simulink model "SF007A_SysFricLrng"  (R2013b)
settings: Solver=FixedStepDiscrete  SolverMode=SingleTasking  StartTime=0.0  StopTime=1  FixedStep=0.002  RelTol=1e-3
PostLoadFcn:
  | , if any(exist('dsrtsu_mdlpostloadfcn', 'file') == [2, 3, 6]), try dsrtsu_mdlpostloadfcn('Execute', bdroot); catch fprintf('Error in PostLoadFcn (dsrtsu_mdlpostloadfcn) for model "%s":\n %s\n', bdroot, lasterr); end, end,
undefined symbols (not defined in the file): ARCHGLBPRM_100MILLISEC_SEC_F32, ARCHGLBPRM_10MILLISEC_SEC_F32, ARCHGLBPRM_180OVERPI_ULS_F32, CONV100MICROSECTOSEC_ULS_F32, FLTINJ_SYSFRICLRNG_SYSFRICOFFS, FricLrngData, HiFricNtc, HWPTNUM_CNT_U08, HWPTNUMSUB1_CNT_U08, HWVELDECDIR_ULS_U08, HWVELINCDIR_ULS_U08, IDXCALCNSCAGFAC_ULS_U08, IDXSELN1_ULS_U08, IDXSELN2_ULS_U08, IDXSELN3_ULS_U08, LRNGENASCAFAC_MILLISEC_U32, NtcSts1, SCAGFACQUARTER_CNT_F32, SCAGFACTEN_CNT_U16, SECIDXSELN_ULS_U08, SysFricLrngBasLineEolFric, SysFricLrngBasLineFric, SysFricLrngBasLineHys, SysFricLrngBasLineRngCntr, SysFricLrngEolFricDifScagFac, SysFricLrngFricChgWght, SysFricLrngFricDiagcThd, SysFricLrngFricDiagcTiThd, SysFricLrngFricHysHwAgPt, SysFricLrngGain, SysFricLrngHwPosnAuthyThd, SysFricLrngHwVelConstrLim, SysFricLrngHwVelHiLim, SysFricLrngHwVelLoLim, SysFricLrngIgnCycFricChgLim, SysFricLrngLatAHiLim, SysFricLrngLatALoLim, SysFricLrngMaskVehSpd, SysFricLrngOperMod1, SysFricLrngRngCntrThd, SysFricLrngThd, SysFricLrngTHiLim, SysFricLrngTLoLim, SysFricLrngVehSpd, SYSFRICOFFSLIM_HWNWTMTR_F32, VEHSPDPTNUM1_ULS_U08, VEHSPDPTNUM2_ULS_U08
libraries: Fil x19, simulink x17, NxtrLim x10, NxtrAbslt x3, NxtrNvM x2, FixdToFloat x2, FloatToFixd x1, LnrIntrpn x1
(part 7 of 7)

== system SF007A_SysFricLrng/SysFricLrng/SysFricLrngPer1/RunningAndCalibrationModes/FricLearning/Calculate Average Friction/Raw Average Calculation/Update LPF/InitAvrgFricLpFil1 ==
  RawAvgFric : Inport
  Action Port : ActionPort  ActionType=case
  CopyRight2 : Subsystem  Description=|  mask(Copyright Information){none=on}
      | Copyright info block.                                               
      |                                                                     
      | Place copyright information at the top of every subsystem in design.
      mask prompts: none "No parameters"
      mask help: Place copyright information at the top of every subsystem in design.
      mask Display:
      | NxtrConf = 'Nexteer Confidential';
      | 
      | sys = bdroot; %handle for the current model ("system")
      | first = get_param(sys,'Created');
      | first = first(end-3:end);  %year is last four digits
      | 
      | last = get_param(sys,'LastModifiedDate');
      | if isempty(last)
      |     last = datestr(now,'yyyy');
      | else
      |     last = last(end-3:end);
      | end
      | 
      | if strcmp(first,last)
      |     fprintf('%s -- Copyright %s Nexteer',NxtrConf,first)
      | else
      |     fprintf('%s -- %s%s- %s Nexteer',NxtrConf,char(169),first,last)
      | end
  FilLpUpdOutp : Subsystem  mask(FilLpUpdOutp){StVar=AvrgFricLpFil1}
      mask prompts: StVar "State Variable:"
      mask help: Simulink implementation of the LPF_OpUpdate_f32_m macro.
      mask init: same as SF007A_SysFricLrng/SysFricLrng/SysFricLrngPer1/RunningAndCalibrationModes/Running Mode/If Action Subsystem/BlendingFricChg/FilLpUpdOutp
      settings: AttributesFormatString=StVar: %<StVar>
      mask Display:
      | port_label('input',1,'Inp')
      | port_label('output',1,'Outp')
      | text(0.2,0.8,'FilLpUpdOutp')
  FiltAvgFric : Outport
  wires:
  RawAvgFric/1 -> FilLpUpdOutp/1(Input)
  FilLpUpdOutp/1(Out1) -> FiltAvgFric/1

== system SF007A_SysFricLrng/SysFricLrng/SysFricLrngPer1/RunningAndCalibrationModes/FricLearning/Calculate Average Friction/Raw Average Calculation/Update LPF/InitAvrgFricLpFil2 ==
  RawAvgFric : Inport
  Action Port : ActionPort  ActionType=case
  CopyRight2 : Subsystem  Description=|  mask(Copyright Information){none=on}
      | Copyright info block.                                               
      |                                                                     
      | Place copyright information at the top of every subsystem in design.
      mask prompts: none "No parameters"
      mask help: Place copyright information at the top of every subsystem in design.
      mask Display:
      | NxtrConf = 'Nexteer Confidential';
      | 
      | sys = bdroot; %handle for the current model ("system")
      | first = get_param(sys,'Created');
      | first = first(end-3:end);  %year is last four digits
      | 
      | last = get_param(sys,'LastModifiedDate');
      | if isempty(last)
      |     last = datestr(now,'yyyy');
      | else
      |     last = last(end-3:end);
      | end
      | 
      | if strcmp(first,last)
      |     fprintf('%s -- Copyright %s Nexteer',NxtrConf,first)
      | else
      |     fprintf('%s -- %s%s- %s Nexteer',NxtrConf,char(169),first,last)
      | end
  FilLpUpdOutp : Subsystem  mask(FilLpUpdOutp){StVar=AvrgFricLpFil2}
      mask prompts: StVar "State Variable:"
      mask help: Simulink implementation of the LPF_OpUpdate_f32_m macro.
      mask init: same as SF007A_SysFricLrng/SysFricLrng/SysFricLrngPer1/RunningAndCalibrationModes/Running Mode/If Action Subsystem/BlendingFricChg/FilLpUpdOutp
      settings: AttributesFormatString=StVar: %<StVar>
      mask Display:
      | port_label('input',1,'Inp')
      | port_label('output',1,'Outp')
      | text(0.2,0.8,'FilLpUpdOutp')
  FiltAvgFric : Outport
  wires:
  RawAvgFric/1 -> FilLpUpdOutp/1(Input)
  FilLpUpdOutp/1(Out1) -> FiltAvgFric/1

== system SF007A_SysFricLrng/SysFricLrng/SysFricLrngPer1/RunningAndCalibrationModes/FricLearning/Calculate Average Friction/Raw Average Calculation/Update LPF/InitAvrgFricLpFil3 ==
  RawAvgFric : Inport
  Action Port : ActionPort  ActionType=case
  CopyRight2 : Subsystem  Description=|  mask(Copyright Information){none=on}
      | Copyright info block.                                               
      |                                                                     
      | Place copyright information at the top of every subsystem in design.
      mask prompts: none "No parameters"
      mask help: Place copyright information at the top of every subsystem in design.
      mask Display:
      | NxtrConf = 'Nexteer Confidential';
      | 
      | sys = bdroot; %handle for the current model ("system")
      | first = get_param(sys,'Created');
      | first = first(end-3:end);  %year is last four digits
      | 
      | last = get_param(sys,'LastModifiedDate');
      | if isempty(last)
      |     last = datestr(now,'yyyy');
      | else
      |     last = last(end-3:end);
      | end
      | 
      | if strcmp(first,last)
      |     fprintf('%s -- Copyright %s Nexteer',NxtrConf,first)
      | else
      |     fprintf('%s -- %s%s- %s Nexteer',NxtrConf,char(169),first,last)
      | end
  FilLpUpdOutp : Subsystem  mask(FilLpUpdOutp){StVar=AvrgFricLpFil3}
      mask prompts: StVar "State Variable:"
      mask help: Simulink implementation of the LPF_OpUpdate_f32_m macro.
      mask init: same as SF007A_SysFricLrng/SysFricLrng/SysFricLrngPer1/RunningAndCalibrationModes/Running Mode/If Action Subsystem/BlendingFricChg/FilLpUpdOutp
      settings: AttributesFormatString=StVar: %<StVar>
      mask Display:
      | port_label('input',1,'Inp')
      | port_label('output',1,'Outp')
      | text(0.2,0.8,'FilLpUpdOutp')
  FiltAvgFric : Outport
  wires:
  RawAvgFric/1 -> FilLpUpdOutp/1(Input)
  FilLpUpdOutp/1(Out1) -> FiltAvgFric/1

== system SF007A_SysFricLrng/SysFricLrng/SysFricLrngPer1/RunningAndCalibrationModes/FricLearning/Calculate Average Friction/Raw Average Calculation/Update LPF/InitAvrgFricLpFil4 ==
  RawAvgFric : Inport
  Action Port : ActionPort  ActionType=default
  CopyRight2 : Subsystem  Description=|  mask(Copyright Information){none=on}
      | Copyright info block.                                               
      |                                                                     
      | Place copyright information at the top of every subsystem in design.
      mask prompts: none "No parameters"
      mask help: Place copyright information at the top of every subsystem in design.
      mask Display:
      | NxtrConf = 'Nexteer Confidential';
      | 
      | sys = bdroot; %handle for the current model ("system")
      | first = get_param(sys,'Created');
      | first = first(end-3:end);  %year is last four digits
      | 
      | last = get_param(sys,'LastModifiedDate');
      | if isempty(last)
      |     last = datestr(now,'yyyy');
      | else
      |     last = last(end-3:end);
      | end
      | 
      | if strcmp(first,last)
      |     fprintf('%s -- Copyright %s Nexteer',NxtrConf,first)
      | else
      |     fprintf('%s -- %s%s- %s Nexteer',NxtrConf,char(169),first,last)
      | end
  FilLpUpdOutp : Subsystem  mask(FilLpUpdOutp){StVar=AvrgFricLpFil4}
      mask prompts: StVar "State Variable:"
      mask help: Simulink implementation of the LPF_OpUpdate_f32_m macro.
      mask init: same as SF007A_SysFricLrng/SysFricLrng/SysFricLrngPer1/RunningAndCalibrationModes/Running Mode/If Action Subsystem/BlendingFricChg/FilLpUpdOutp
      settings: AttributesFormatString=StVar: %<StVar>
      mask Display:
      | port_label('input',1,'Inp')
      | port_label('output',1,'Outp')
      | text(0.2,0.8,'FilLpUpdOutp')
  FiltAvgFric : Outport
  wires:
  RawAvgFric/1 -> FilLpUpdOutp/1(Input)
  FilLpUpdOutp/1(Out1) -> FiltAvgFric/1

== system SF007A_SysFricLrng/SysFricLrng/SysFricLrngPer1/RunningAndCalibrationModes/FricLearning/Range Counter Manager/Range Counter Control1/UpdateBaselineFric/CopyRight2 ==

== system SF007A_SysFricLrng/SysFricLrng/SysFricLrngPer1/RunningAndCalibrationModes/FricLearning/Range Counter Manager/Range Counter Threshold Calculation/Do Nothig/CopyRight2 ==

== system SF007A_SysFricLrng/SysFricLrng/SysFricLrngPer1/RunningAndCalibrationModes/FricLearning/Range Counter Manager/Range Counter Threshold Calculation/RangeCounterThreshExceeded/CopyRight2 ==

== system SF007A_SysFricLrng/SysFricLrng/SysFricLrngPer1/RunningAndCalibrationModes/LearningConstraint/ColTqconstraint/ColTqAryCalcn/12 Delay's Execution/CopyRight2 ==

== system SF007A_SysFricLrng/SysFricLrng/SysFricLrngPer1/RunningAndCalibrationModes/LearningConstraint/HwAngConstraint/Handwheel Angle Buffer/12 Delay's Execution/CopyRight2 ==

== system SF007A_SysFricLrng/SysFricLrng/SysFricLrngPer1/RunningAndCalibrationModes/LearningConstraint/HwVelConstraint/Handwheel Velocity Buffer/12 Delay's Execution/CopyRight2 ==

== system SF007A_SysFricLrng/SysFricLrng/SysFricLrngPer1/RunningAndCalibrationModes/LearningConstraint/HwVelConstraint/Range_Monotonicity Calculation/ AllGTZ/CopyRight2 ==

== system SF007A_SysFricLrng/SysFricLrng/SysFricLrngPer1/RunningAndCalibrationModes/LearningConstraint/HwVelConstraint/Range_Monotonicity Calculation/AllLTZ/CopyRight2 ==

== system SF007A_SysFricLrng/SysFricLrng/SysFricLrngPer1/RunningAndCalibrationModes/LearningConstraint/VehSpdConstraint/VehSpdIdxCalcn/If Action Subsystem/CopyRight2 ==

== system SF007A_SysFricLrng/SysFricLrng/SysFricLrngPer1/RunningAndCalibrationModes/LearningConstraint/VehSpdConstraint/VehSpdIdxCalcn/If Action Subsystem1/CopyRight2 ==

== system SF007A_SysFricLrng/SysFricLrng/SysFricLrngPer1/RunningAndCalibrationModes/FricLearning/Calculate Average Friction/NTC FAIL/GetTiSpan100MicroSec32bit/No wrapping/CopyRight2 ==

== system SF007A_SysFricLrng/SysFricLrng/SysFricLrngPer1/RunningAndCalibrationModes/FricLearning/Calculate Average Friction/NTC FAIL/GetTiSpan100MicroSec32bit/Wrapping/CopyRight2 ==

== system SF007A_SysFricLrng/SysFricLrng/SysFricLrngPer1/RunningAndCalibrationModes/FricLearning/Calculate Average Friction/NTC FAIL/NTCFAIL/SetNtcSts/SetNtcSts ==
  note: Note:
      |
      | - "ISO Fault Debounce Design" Simulink block intent to use here for Simulation purpose only. Do not Code this block
  NtcNr : Inport
  NtcStInfo : Inport  Port=2
  NtcSts : Inport  Port=3
  DebStep : Inport  Port=4
  CopyRight2 : Subsystem  Description=|  mask(Copyright Information){none=on}
      | Copyright info block.                                               
      |                                                                     
      | Place copyright information at the top of every subsystem in design.
      mask prompts: none "No parameters"
      mask help: Place copyright information at the top of every subsystem in design.
      mask Display:
      | NxtrConf = 'Nexteer Confidential';
      | 
      | sys = bdroot; %handle for the current model ("system")
      | first = get_param(sys,'Created');
      | first = first(end-3:end);  %year is last four digits
      | 
      | last = get_param(sys,'LastModifiedDate');
      | if isempty(last)
      |     last = datestr(now,'yyyy');
      | else
      |     last = last(end-3:end);
      | end
      | 
      | if strcmp(first,last)
      |     fprintf('%s -- Copyright %s Nexteer',NxtrConf,first)
      | else
      |     fprintf('%s -- %s%s- %s Nexteer',NxtrConf,char(169),first,last)
      | end
  Data Store Write : DataStoreWrite  DataStoreName=Ntc0X0A2Qlfr
  Data Type Conversion4 : DataTypeConversion  OutDataTypeStr=Enum: SigQlfr1
  Ground : Ground
  ISO Fault Debounce Design : Stateflow chart  TreatAsAtomicUnit=on
      settings: AttributesFormatString=|
      | Simulation Purpose Only.
      | Do Not Code this block
      | Diagnostic Manager Owns this requirement
  Terminator : Terminator
  Terminator1 : Terminator
  wires:
  NtcStInfo/1 -> Terminator1/1
  NtcNr/1 -> Terminator/1
  DebStep/1 -> ISO Fault Debounce Design/2(DebStep)
  ISO Fault Debounce Design/1(Qualifier) -> Data Type Conversion4/1
  Ground/1 -> ISO Fault Debounce Design/3(SvcClr)
  Data Type Conversion4/1 -> Data Store Write/1
  NtcSts/1 -> ISO Fault Debounce Design/1(NtcSts)

== system SF007A_SysFricLrng/SysFricLrng/SysFricLrngPer1/RunningAndCalibrationModes/FricLearning/Calculate Average Friction/NTC PASS /SetNtcSts/SetNtcSts/CopyRight2 ==

== system SF007A_SysFricLrng/SysFricLrng/SysFricLrngPer1/RunningAndCalibrationModes/FricLearning/Calculate Average Friction/Raw Average Calculation/Update LPF/InitAvrgFricLpFil1/CopyRight2 ==

== system SF007A_SysFricLrng/SysFricLrng/SysFricLrngPer1/RunningAndCalibrationModes/FricLearning/Calculate Average Friction/Raw Average Calculation/Update LPF/InitAvrgFricLpFil1/FilLpUpdOutp ==
  Input : Inport
  Add : Sum
  Data Store Read : DataStoreRead  DataStoreName=AvrgFricLpFil1  DataStoreElements=AvrgFricLpFil1.FilSt#AvrgFricLpFil1.FilGain
  Data Store Write : DataStoreWrite  DataStoreName=AvrgFricLpFil1  DataStoreElements=AvrgFricLpFil1.FilSt
  Display1 : Display
  Display2 : Display
  Product : Product
  Subtract : Sum  Inputs=+-
  Out1 : Outport  OutDataTypeStr=single
  wires:
  Data Store Read/2 -> Display1/1, Product/2
  Add/1 -> Out1/1, Data Store Write/1
  Product/1 -> Add/2
  Subtract/1 -> Product/1
  Input/1 -> Subtract/1
  Data Store Read/1 -> Display2/1, Subtract/2, Add/1

== system SF007A_SysFricLrng/SysFricLrng/SysFricLrngPer1/RunningAndCalibrationModes/FricLearning/Calculate Average Friction/Raw Average Calculation/Update LPF/InitAvrgFricLpFil2/CopyRight2 ==

== system SF007A_SysFricLrng/SysFricLrng/SysFricLrngPer1/RunningAndCalibrationModes/FricLearning/Calculate Average Friction/Raw Average Calculation/Update LPF/InitAvrgFricLpFil2/FilLpUpdOutp ==
  Input : Inport
  Add : Sum
  Data Store Read : DataStoreRead  DataStoreName=AvrgFricLpFil2  DataStoreElements=AvrgFricLpFil2.FilSt#AvrgFricLpFil2.FilGain
  Data Store Write : DataStoreWrite  DataStoreName=AvrgFricLpFil2  DataStoreElements=AvrgFricLpFil2.FilSt
  Display1 : Display
  Display2 : Display
  Product : Product
  Subtract : Sum  Inputs=+-
  Out1 : Outport  OutDataTypeStr=single
  wires:
  Data Store Read/2 -> Display1/1, Product/2
  Add/1 -> Out1/1, Data Store Write/1
  Product/1 -> Add/2
  Subtract/1 -> Product/1
  Input/1 -> Subtract/1
  Data Store Read/1 -> Display2/1, Subtract/2, Add/1

== system SF007A_SysFricLrng/SysFricLrng/SysFricLrngPer1/RunningAndCalibrationModes/FricLearning/Calculate Average Friction/Raw Average Calculation/Update LPF/InitAvrgFricLpFil3/CopyRight2 ==

== system SF007A_SysFricLrng/SysFricLrng/SysFricLrngPer1/RunningAndCalibrationModes/FricLearning/Calculate Average Friction/Raw Average Calculation/Update LPF/InitAvrgFricLpFil3/FilLpUpdOutp ==
  Input : Inport
  Add : Sum
  Data Store Read : DataStoreRead  DataStoreName=AvrgFricLpFil3  DataStoreElements=AvrgFricLpFil3.FilSt#AvrgFricLpFil3.FilGain
  Data Store Write : DataStoreWrite  DataStoreName=AvrgFricLpFil3  DataStoreElements=AvrgFricLpFil3.FilSt
  Display1 : Display
  Display2 : Display
  Product : Product
  Subtract : Sum  Inputs=+-
  Out1 : Outport  OutDataTypeStr=single
  wires:
  Data Store Read/2 -> Display1/1, Product/2
  Add/1 -> Out1/1, Data Store Write/1
  Product/1 -> Add/2
  Subtract/1 -> Product/1
  Input/1 -> Subtract/1
  Data Store Read/1 -> Display2/1, Subtract/2, Add/1

== system SF007A_SysFricLrng/SysFricLrng/SysFricLrngPer1/RunningAndCalibrationModes/FricLearning/Calculate Average Friction/Raw Average Calculation/Update LPF/InitAvrgFricLpFil4/CopyRight2 ==

== system SF007A_SysFricLrng/SysFricLrng/SysFricLrngPer1/RunningAndCalibrationModes/FricLearning/Calculate Average Friction/Raw Average Calculation/Update LPF/InitAvrgFricLpFil4/FilLpUpdOutp ==
  Input : Inport
  Add : Sum
  Data Store Read : DataStoreRead  DataStoreName=AvrgFricLpFil4  DataStoreElements=AvrgFricLpFil4.FilSt#AvrgFricLpFil4.FilGain
  Data Store Write : DataStoreWrite  DataStoreName=AvrgFricLpFil4  DataStoreElements=AvrgFricLpFil4.FilSt
  Display1 : Display
  Display2 : Display
  Product : Product
  Subtract : Sum  Inputs=+-
  Out1 : Outport  OutDataTypeStr=single
  wires:
  Data Store Read/2 -> Display1/1, Product/2
  Add/1 -> Out1/1, Data Store Write/1
  Product/1 -> Add/2
  Subtract/1 -> Product/1
  Input/1 -> Subtract/1
  Data Store Read/1 -> Display2/1, Subtract/2, Add/1

== system SF007A_SysFricLrng/SysFricLrng/SysFricLrngPer1/RunningAndCalibrationModes/FricLearning/Calculate Average Friction/NTC FAIL/NTCFAIL/SetNtcSts/SetNtcSts/CopyRight2 ==
